simulink model "lab6_heater"  (Simulink 10.2)
settings: Solver=ode15s  StartTime=0.0  StopTime=7200  RelTol=1e-6
settings Model: Creator=mluser  LastModifiedBy=avi  MultiThreadCoSim=auto
settings DataIOCC: SaveFormat=Dataset  SignalLoggingSaveFormat=Dataset  ReturnWorkspaceOutputs=on  Refine=4
settings OptimizationCC: LifeSpan=auto
settings DebuggingCC: UnderspecifiedInitializationDetection=Simplified  MergeDetectMultiDrivingBlocksExec=error  FcnCallInpInsideContextMsg=error  SFUnexpectedBacktrackingDiag=error  SFNoUnconditionalDefaultTransitionDiag=error  SFExecutionAtInitializationDiag=warning  SFMachineParentedDataDiag=error  ArithmeticOperatorsInVariantConditions=error
settings HardwareCC: ProdBitPerPointer=64  ProdBitPerSizeT=64  ProdBitPerPtrDiffT=64  ProdLargestAtomicFloat=Float  ProdIntDivRoundTo=Zero  ProdEndianess=LittleEndian  ProdWordSize=64  ProdHWDeviceType=Intel->x86-64 (Windows64)
settings ModelReferenceCC: PropagateSignalLabelsOutOfModel=on
settings SFSimCC: SimUseLocalCustomCode=on  CustomCodeUndefinedFunction=FilterOut
settings RTWCC: RTWUseLocalCustomCode=on
settings CodeAppCC: StateflowObjectComments=off
settings GRTTargetCC: TargetLangStandard=C99 (ISO)  CombineOutputUpdateFcns=on  GRTInterface=off
settings ConfigComp: CovMetricSettings=dwe  CovSaveCumulativeToWorkspaceVar=off  CovSaveSingleToWorkspaceVar=off  CovExternalEMLEnable=on

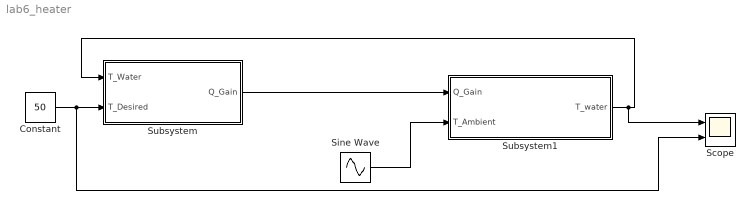
== system lab6_heater ==
  Constant : Constant  Value=50
  Scope : Scope  NumInputPorts=2
  Sine Wave : Sin  Amplitude=10  Bias=25  Frequency=.00005  SampleTime=0
  Subsystem : Subsystem
  Subsystem1 : Subsystem
  wires:
  Subsystem1/1(T_water) -> Scope/1, Subsystem/1(T_Water)
  Constant/1 -> Scope/2, Subsystem/2(T_Desired)
  Subsystem/1(Q_Gain) -> Subsystem1/1(Q_Gain)
  Sine Wave/1 -> Subsystem1/2(T_Ambient)

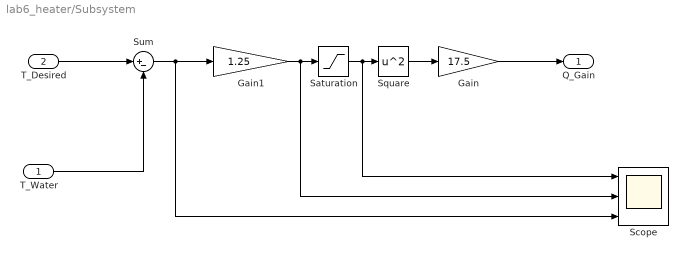
== system lab6_heater/Subsystem ==
  T_Water : Inport
  T_Desired : Inport  Port=2
  Gain : Gain  Gain=17.5
  Gain1 : Gain  Gain=1.25
  Saturation : Saturate  UpperLimit=15  LowerLimit=0
  Scope : Scope  NumInputPorts=3
  Square : Math  Operator=square  SaturateOnIntegerOverflow=on
  Sum : Sum  Inputs=|+-
  Q_Gain : Outport
  wires:
  Saturation/1 -> Scope/1, Square/1
  Sum/1 -> Scope/3, Gain1/1
  T_Desired/1 -> Sum/1
  T_Water/1 -> Sum/2
  Gain/1 -> Q_Gain/1
  Gain1/1 -> Scope/2, Saturation/1
  Square/1 -> Gain/1

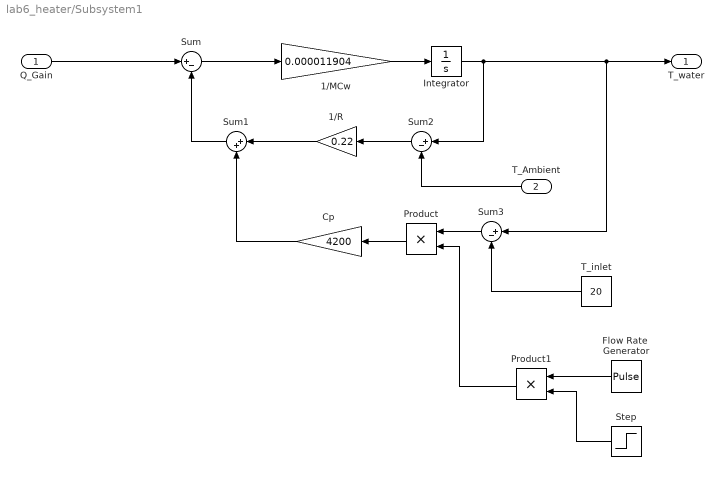
== system lab6_heater/Subsystem1 ==
  Q_Gain : Inport
  T_Ambient : Inport  Port=2
  1/MCw : Gain  Gain=0.000011904
  1/R : Gain  Gain=0.22
  Cp : Gain  Gain=4200
  Flow Rate  Generator : DiscretePulseGenerator  PulseType=Time based  Amplitude=1/60  Period=300  PulseWidth=60  PhaseDelay=2500
  Integrator : Integrator  InitialCondition=20
  Product : Product
  Product1 : Product
  Step : Step  Time=2500  SampleTime=0
  Sum : Sum  Inputs=|+-
  Sum1 : Sum  Inputs=|++
  Sum2 : Sum  Inputs=|+-
  Sum3 : Sum  Inputs=|+-
  T_inlet : Constant  Value=20
  T_water : Outport
  wires:
  Sum2/1 -> 1/R/1
  Sum3/1 -> Product/1
  1/R/1 -> Sum1/1
  Cp/1 -> Sum1/2
  Flow Rate  Generator/1 -> Product1/1
  1/MCw/1 -> Integrator/1
  Sum/1 -> 1/MCw/1
  T_inlet/1 -> Sum3/2
  Sum1/1 -> Sum/2
  Product/1 -> Cp/1
  Integrator/1 -> Sum2/1, T_water/1, Sum3/1
  T_Ambient/1 -> Sum2/2
  Product1/1 -> Product/2
  Step/1 -> Product1/2
  Q_Gain/1 -> Sum/1
